simulink subsystem "Driver_Input"  (R2021b)
settings: Solver=VariableStepAuto  StartTime=0.0  StopTime=10.0  RelTol=1e-3
PostLoadFcn:
  | if any(exist('dsrtsu_mdlpostloadfcn', 'file') ~= 0), dsrtsu_mdlpostloadfcn('Execute', bdroot); end
libraries: simulink x9, dspstat3 x7, rtican x3, rti1401lib_adc_type4 x1
(part 1 of 2)
settings Model: DSRTSU_INTERNAL_RTI_VER=530  DSRTSU_INTERNAL_RTI_TYPE=rti1401  RTICANMMDATA=struct('GeneralSetupData',struct('modelroot','C:\Users\FEM\Documents\MATLAB\VCM_VehicleDynamicSim\VCMProgram\IO','generalsettings',struct('filesettings',struct('destfolder',struct('Name','RTICANMM_FILES','Check',1),'buildfolder',struct('Name','.','Check',1),'AbsDestfolder',struct('Name','C:\Users\FEM\Documents\MATLAB\VCM_VehicleDynamicSim\VCMProgram\IO\RTICANMM_FILES'),'AbsBuildfolder',struct('Name','C:\Users\FEM\Documents\MATLAB\VCM_VehicleDynamicSim\VCMProgram\IO'))),'options',struct('addpaths',1,'rmpaths',1,'addtrcexclusion',logical(1),'cannavigator',struct('checkmonitoring',0),'show_usrtrc',0,'use_usrtrc',0),'advanced',struct('options',ones(1,100)),'MPSetup',{{}},'RTI',struct('Type','GRT','Ver','','Date',''),'modelname','Driver_Input','block','Driver_Input'))  Creator=tsuyoshi  LastModifiedBy=FEM

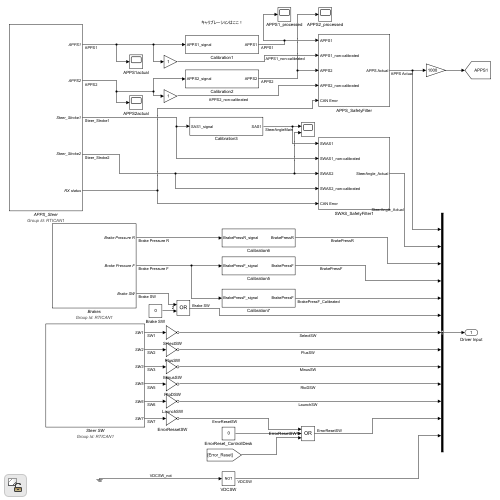
[thumbnail: Simulink's stored preview of the top-level diagram]
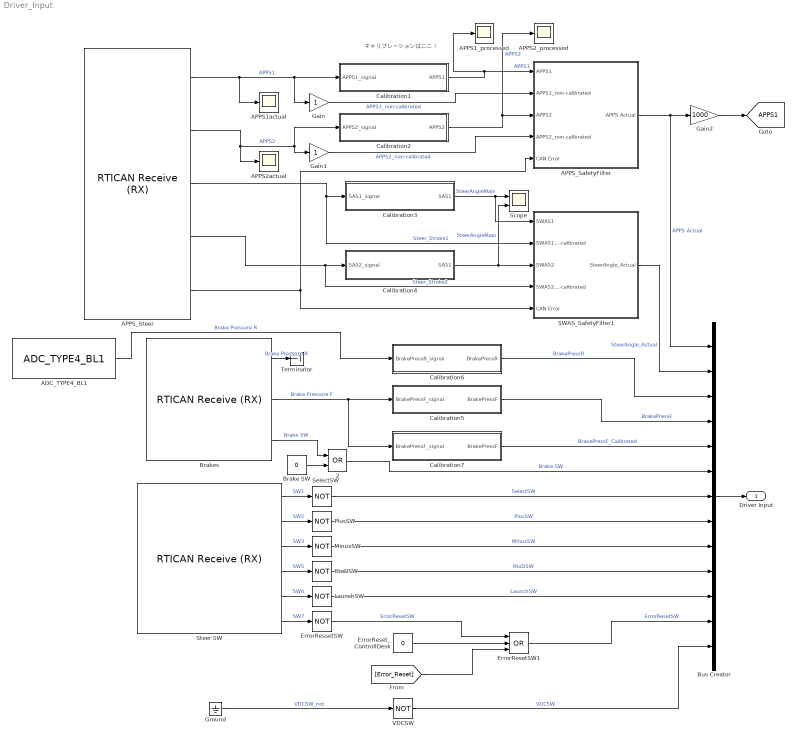
== system Driver_Input ==
  note: キャリブレーションはここ！
  2 : Logic  Operator=OR  AllPortsSameDT=off  OutDataTypeStr=boolean
  ADC_TYPE4_BL1 : rti1401lib_adc_type4/ADC_TYPE4_BL1  DSProperties=struct('RTI',struct('Version',uint32(2),'BlockType',struct('isSLSource',uint8(1),'isSLSink',uint8(1),'isHWSource',uint8(0),'isHWSink',uint8(1),'isSetup',uint8(0),'isInline',uint8(1),'isNonInline',uint8(0),'isInterrupt',uint8(0),'isChannelwise',uint8(1)),'IOBoardType',{{'DS1401','STD','ADCT4'}},'UnitType','ADC','Identifier','ADC','DialogType','ML','BlockSet','NONE','SlaveProcessor','NONE'))  RTIBlockInterface=struct('InputPortsActive',0,'InputPortsWidth',int32(1),'InputPortsDataType',{{'SS_BOOLEAN'}},'InputPortsName',{{'Continue'}},'OutputPortsActive',[1 0],'OutputPortsWidth',int32([1 1]),'OutputPortsDataType',{{'SS_DOUBLE','SS_UINT8'}},'OutputPortsName',{{'ADC','Status'}},'DialogFcn','rti1401stdadct4adcgui','SampleTime',{{-1}},'InitLevel',3,'IconTransparency','on','BlockDisplay',{{['ADC TP4\nModule: 1\nChannel: 6'],'center'}},'BlockName',struct('Token',{{'ADC_TYPE4_BL1'}}))  RTIBlockParameters=struct('ADCSWStartDisable',{{0,'OFF',[0 1]}},'ModuleNo',{{1,'OFF',[1 16]}},'ChannelNo',{{6,'OFF',[1 16]}},'ConversionMode',{{1,'OFF',[1 2]}},'SampleMode',{{1,'OFF',[1 2]}},'TriggerSource',{{1,'OFF',[1 5]}},'EdgePolarity',{{1,'OFF',[1 2]}},'ConversionTriggerSource',{{2,'OFF',[1 6]}},'ConversionEdgePolarity',{{1,'OFF',[1 2]}},'ConversionPeriod',{{'1e-06','OFF',[]}},'ConversionPeriodCheck',{{0,'OFF',[]}},'BurstTriggerSource',{{1,'OFF',[1 6]}},'BurstEdgePolarity',{{1,'OFF',[1 2]}},'BurstSize',{{'10','OFF',[]}},'BurstSizeCheck',{{0,'OFF',[]}},'DataSetOffset',{{'0','OFF',[]}},'DataSetOffsetCheck',{{0,'OFF',[]}},'DataSetLength',{{'1','OFF',[]}},'DataSetLengthCheck',{{0,'OFF',[]}},'ReadMode',{{1,'OFF',[1 2]}},'SampleTime',{{'-1','OFF',[-1 inf]}},'SampleTimeCheck',{{1,'OFF',[]}},'StatusPortEnable',{{0,'OFF',[0 1]}},'VoltageRange',{{2,'OFF',[1 2]}},'TLCFileName',{{'rti1401adc_t4_adc','OFF',[]}})  RTISFcnParameters=struct('ADCSWStartDisable','int32','ModuleNo','int32','ChannelNo','int16','ConversionMode','int16','SampleMode','int16','TriggerSource','int16','EdgePolarity','int16','ConversionTriggerSource','int16','ConversionEdgePolarity','int16','ConversionPeriod','double','BurstTriggerSource','int16','BurstEdgePolarity','int16','BurstSize','int16','DataSetOffset','int16','DataSetLength','int16','ReadMode','int16','SampleTime','double','StatusPortEnable','int16','VoltageRange','int16','TLCFileName','char')  RTIBlockParaDefault=struct('ADCSWStartDisable',0,'ModuleNo',1,'ChannelNo',1,'ConversionMode',1,'SampleMode',1,'TriggerSource',1,'EdgePolarity',1,'ConversionTriggerSource',2,'ConversionEdgePolarity',1,'ConversionPeriod',1e-6,'ConversionPeriodCheck',0,'BurstTriggerSource',1,'BurstEdgePolarity',1,'BurstSize',10,'BurstSizeCheck',0,'DataSetOffset',0,'DataSetOffsetCheck',0,'DataSetLength',1,'DataSetLengthCheck',0,'ReadMode',1,'SampleTime',-1,'SampleTimeCheck',1,'StatusPortEnable',0,'VoltageRange',1,'TLCFileName','rti1401adc_t4_adc')
  APPS1_processed : Scope
  APPS1actual : Scope
  APPS2_processed : Scope
  APPS2actual : Scope
  APPS_SafetyFilter : Subsystem
  APPS_Steer : rtican/RTICAN Receive (RX)   Reserved1=[]  Reserved2=[]  Reserved3=[]  Reserved4=[]  SfcnMessage=[]  Msg_Struct=[]  BoardTypeNo=[]  BoardNo=[]  ChannelNo=[]  Parameters=[]  DialogFcn=[]  UnitName=[]  Revision=[]  UnitValues=[]  DSProperties=struct('RTI',struct('Version',uint32(5),'BlockType',struct('isSLSource',uint8(1),'isSLSink',uint8(1),'isHWSource',uint8(0),'isHWSink',uint8(0),'isSetup',uint8(0),'isInline',uint8(1),'isNonInline',uint8(0),'isInterrupt',uint8(0),'isChannelwise',uint8(0)),'IOBoardType','RTICAN','UnitType','MESSAGE','Identifier','RX','DialogType','MSVC','BlockSet','RTICAN','SlaveProcessor','CAN'))  RTIBlockInterface=struct('OutputPortsWidth',int32([1 1 1 1 1]),'OutputPortsActive',[1 1 1 1 1],'OutputPortsName',{{'APPS1','APPS2','Steer_Stroke1','Steer_Stroke2',['RX status']}},'OutputPortsDataType',{{'SS_DOUBLE','SS_DOUBLE','SS_DOUBLE','SS_DOUBLE','SS_DOUBLE'}},'OutputPortsLabel',{{'APPS1','APPS2','Steer_Stroke1','Steer_Stroke2',''}},'OutputPortsLabelMode','ON','InputPortsWidth',int32(0),'InputPortsActive',0,'DialogFcn','rtican_message_interface_gui','BlockDisplay',{{'','center'}},'IconTransparency','on','ParameterTunableNames',{{}},'InitLevel',3,'BlockName',struct('Token',{{'APPS_Steer'}}),'SampleTime',{{0.01}},'TriggerPort',{{'none'}},'EnablePort',{{'none'}})  RTIBlockParameters=struct('BoardTypeNo',{{1,'OFF',[]}},'BoardNo',{{1,'ON',[1 16]}},'ChannelNo',{{1,'ON',[1 2]}},'Parameters',{{struct('DataFileSupport',struct('DataFileSelectedMaster',0,'DataFileSelectedLocal',0,'DataFileName',['<no datafile support>|'],'DataFileDate','','SelectedFile',['<no file selected>']),'Options',struct('StatusSelected',1,'TimeSelected',0,'DeltaTimeSelected',0,'BytePortSelected',0,'MessageLengthSelected',0,'TriggerPort',struct('Selected',0,'TriggerType',0),'UserCoding',struct('Selected',0,'InterfaceFile','UserDecodingFile','FcnName','UserDecodeFcn','InportSelected',0,'InportWidth',1,'OutportSelected',0,'OutportWidth',1),'EnablePortSelected',0,'SignalOnPortnameSelected',1,'UseRXService',0),'Message',struct('MsgOnBlocknameSelected',1,'MsgName','APPS_Steer','MsgIdFormat',0,'MsgId',513,'MsgLength',8,'NumSignals',4,'SampleTime',0.01,'Signal',struct('SgnName',{'APPS1','APPS2','Steer_Stroke1','Steer_Stroke2'},'SgnStartBit',{0,16,32,48},'SgnLength',{16,16,16,16},'SgnType',{0,0,0,0},'ModeValue',{-1,-1,-1,-1},'DataType',{0,0,0,0},'ByteLayout',{0,0,0,0},'Factor',{1,1,1,1},'Offset',{0,0,0,0},'SgnComment',{{''},{''},{''},{''}},'SgnUnit',{'','','',''},'Min',{0,0,0,0},'Max',{0,0,0,0},'SLDataType',{'SS_DOUBLE','SS_DOUBLE','SS_DOUBLE','SS_DOUBLE'}),'MsgIdNumFormat',1,'MsgComment',{{''}}),'Version',1.2,'general',struct('isFromLib',0)),'OFF',[]}},'GroupId',{{struct('Group',{{'RTICAN'}},'No',1,'Behavior',{{'NAMECHANGE'}},'BlockType',{{'SINK'}},'NameChangeFlag',0),'OFF',[]}},'SFcnRTICANMessage',{{struct('MsgType','RX','SFcnPortType','Scalar','MsgName','APPS_Steer','MsgIdFormat','STD','MsgId',513,'MsgLength',8,'NumSignals',4,'SampleTime',0.01,'Signal',struct('SgnName',{'APPS1','APPS2','Steer_Stroke1','Steer_Stroke2'},'SgnStartBit',{0,16,32,48},'SgnLength',{16,16,16,16},'SgnType',{'standard','standard','standard','standard'},'ModeValue',{-1,-1,-1,-1},'DataType',{['unsigned int'],['unsigned int'],['unsigned int'],['unsigned int']},'ByteLayout',{['little endian'],['little endian'],['little endian'],['little endian']},'Factor',{1,1,1,1},'Offset',{0,0,0,0},'SLDataType',{'SS_DOUBLE','SS_DOUBLE','SS_DOUBLE','SS_DOUBLE'}),'StatusSelected','yes','TimeSelected','no','DeltaTimeSelected','no','BytePortSelected','no','MessageLengthSelected','no','TriggerPort',struct('Selected','no','TriggerType',0),'UserCoding',struct('Selected','no','InterfaceFile','UserDecodingFile','FcnName','UserDecodeFcn','InportSelected','no','InportWidth',1,'OutportSelected','no','OutportWidth',1),'EnablePortSelected','no','UseRXService','no','BoardType','DS1','BoardNo',1,'ControllerNo',1),'OFF',[]}},'TLCFileName',{{'rtican_rx_message','OFF',[]}})  RTISFcnParameters=struct('SFcnRTICANMessage','struct','TLCFileName','char')  RTIBlockParaDefault=struct('BoardTypeNo',4302,'BoardNo',1,'ChannelNo',1,'Parameters',struct('DataFileSupport',struct('DataFileSelectedMaster',0,'DataFileSelectedLocal',0,'DataFileName','','DataFileDate','','SelectedFile',['<no file selected>']),'Options',struct('StatusSelected',1,'TimeSelected',1,'DeltaTimeSelected',1,'BytePortSelected',0,'MessageLengthSelected',0,'TriggerPort',struct('Selected',0,'TriggerType','rising'),'UserCoding',struct('Selected',0,'InterfaceFile','UserDecodingFile','FcnName','UserDecodeFcn','InportSelected',0,'InportWidth',1,'OutportSelected',0,'OutportWidth',1),'EnablePortSelected',0,'SignalOnPortnameSelected',1,'UseRXService',0),'Message',struct('MsgOnBlocknameSelected',0,'MsgName',['RX Message'],'MsgIdFormat',0,'MsgId',100,'MsgLength',8,'NumSignals',1,'SampleTime',-1,'Signal',struct('SgnName',['RX signal'],'SgnStartBit',0,'SgnLength',8,'SgnType',0,'ModeValue',-1,'DataType',0,'SLDataType','SS_DOUBLE','ByteLayout',0,'Factor',1,'Offset',0,'Min',0,'Max',255,'SgnComment',{{}},'SgnUnit',''),'MsgIdNumFormat',0,'MsgComment',{{''}}),'Version',1.2,'general',struct('isFromLib',1)),'GroupId',struct('Group',{{'RTICAN'}},'No',1,'Behavior',{{'NAMECHANGE'}},'BlockType',{{'SINK'}},'NameChangeFlag',0),'SFcnRTICANMessage',struct('MsgType','RX','MsgName',['RX Message'],'MsgIdFormat','STD','MsgId',100,'MsgLength',8,'NumSignals',1,'SampleTime',-1,'Signal',struct('SgnName',['RX signal'],'SgnStartBit',0,'SgnLength',8,'SgnType','standard','ModeValue',-1,'DataType',['unsigned int'],'ByteLayout',['little endian'],'SLDataType','SS_DOUBLE','Factor',1,'Offset',0),'StatusSelected','yes','TimeSelected','yes','DeltaTimeSelected','yes','BytePortSelected','no','MessageLengthSelected','no','EnablePortSelected','no','UserCoding',struct('Selected','no','InterfaceFile','UserDecodingFile','FcnName','UserDecodeFcn','InportSelected','no','InportWidth',1,'OutportSelected','no','OutportWidth',1),'TriggerPort',struct('Selected','no','TriggerType','rising'),'UseRXService','no','BoardType','DS4302','BoardNo',1,'ControllerNo',1,'SFcnPortType','Scalar'),'TLCFileName','rtican_rx_message')
      settings: AttributesFormatString=Group Id: RTICAN1\n  SourceProductName=dSPACE RTI CAN Blockset
  Brake SW : Constant  Value=0
  Brakes : rtican/RTICAN Receive (RX)   Reserved1=[]  Reserved2=[]  Reserved3=[]  Reserved4=[]  SfcnMessage=[]  Msg_Struct=[]  BoardTypeNo=[]  BoardNo=[]  ChannelNo=[]  Parameters=[]  DialogFcn=[]  UnitName=[]  Revision=[]  UnitValues=[]  DSProperties=struct('RTI',struct('Version',uint32(5),'BlockType',struct('isSLSource',uint8(1),'isSLSink',uint8(1),'isHWSource',uint8(0),'isHWSink',uint8(0),'isSetup',uint8(0),'isInline',uint8(1),'isNonInline',uint8(0),'isInterrupt',uint8(0),'isChannelwise',uint8(0)),'IOBoardType','RTICAN','UnitType','MESSAGE','Identifier','RX','DialogType','MSVC','BlockSet','RTICAN','SlaveProcessor','CAN'))  RTIBlockInterface=struct('OutputPortsWidth',int32([1 1 1]),'OutputPortsActive',[1 1 1],'OutputPortsName',{{['Brake Pressure R'],['Brake Pressure F'],['Brake SW']}},'OutputPortsDataType',{{'SS_DOUBLE','SS_DOUBLE','SS_DOUBLE'}},'OutputPortsLabel',{{['Brake Pressure R'],['Brake Pressure F'],['Brake SW']}},'OutputPortsLabelMode','ON','InputPortsWidth',int32(0),'InputPortsActive',0,'DialogFcn','rtican_message_interface_gui','BlockDisplay',{{'','center'}},'IconTransparency','on','ParameterTunableNames',{{}},'InitLevel',3,'BlockName',struct('Token',{{'Brakes'}}),'SampleTime',{{0.01}},'TriggerPort',{{'none'}},'EnablePort',{{'none'}})  RTIBlockParameters=struct('BoardTypeNo',{{1,'OFF',[]}},'BoardNo',{{1,'ON',[1 16]}},'ChannelNo',{{1,'ON',[1 2]}},'Parameters',{{struct('DataFileSupport',struct('DataFileSelectedMaster',0,'DataFileSelectedLocal',0,'DataFileName',['<no datafile support>|'],'DataFileDate','','SelectedFile',['<no file selected>']),'Options',struct('StatusSelected',0,'TimeSelected',0,'DeltaTimeSelected',0,'BytePortSelected',0,'MessageLengthSelected',0,'TriggerPort',struct('Selected',0,'TriggerType',0),'UserCoding',struct('Selected',0,'InterfaceFile','UserDecodingFile','FcnName','UserDecodeFcn','InportSelected',0,'InportWidth',1,'OutportSelected',0,'OutportWidth',1),'EnablePortSelected',0,'SignalOnPortnameSelected',1,'UseRXService',0),'Message',struct('MsgOnBlocknameSelected',1,'MsgName','Brakes','MsgIdFormat',0,'MsgId',514,'MsgLength',8,'NumSignals',3,'SampleTime',0.01,'Signal',struct('SgnName',{['Brake Pressure R'],['Brake Pressure F'],['Brake SW']},'SgnStartBit',{0,16,32},'SgnLength',{16,16,8},'SgnType',{0,0,0},'ModeValue',{-1,-1,-1},'DataType',{0,0,0},'ByteLayout',{0,0,0},'Factor',{1,1,1},'Offset',{0,0,0},'SgnComment',{{''},{''},{''}},'SgnUnit',{'','',''},'Min',{0,0,0},'Max',{0,0,0},'SLDataType',{'SS_DOUBLE','SS_DOUBLE','SS_DOUBLE'}),'MsgIdNumFormat',1,'MsgComment',{{''}}),'Version',1.2,'general',struct('isFromLib',0)),'OFF',[]}},'GroupId',{{struct('Group',{{'RTICAN'}},'No',1,'Behavior',{{'NAMECHANGE'}},'BlockType',{{'SINK'}},'NameChangeFlag',0),'OFF',[]}},'SFcnRTICANMessage',{{struct('MsgType','RX','SFcnPortType','Scalar','MsgName','Brakes','MsgIdFormat','STD','MsgId',514,'MsgLength',8,'NumSignals',3,'SampleTime',0.01,'Signal',struct('SgnName',{['Brake Pressure R'],['Brake Pressure F'],['Brake SW']},'SgnStartBit',{0,16,32},'SgnLength',{16,16,8},'SgnType',{'standard','standard','standard'},'ModeValue',{-1,-1,-1},'DataType',{['unsigned int'],['unsigned int'],['unsigned int']},'ByteLayout',{['little endian'],['little endian'],['little endian']},'Factor',{1,1,1},'Offset',{0,0,0},'SLDataType',{'SS_DOUBLE','SS_DOUBLE','SS_DOUBLE'}),'StatusSelected','no','TimeSelected','no','DeltaTimeSelected','no','BytePortSelected','no','MessageLengthSelected','no','TriggerPort',struct('Selected','no','TriggerType',0),'UserCoding',struct('Selected','no','InterfaceFile','UserDecodingFile','FcnName','UserDecodeFcn','InportSelected','no','InportWidth',1,'OutportSelected','no','OutportWidth',1),'EnablePortSelected','no','UseRXService','no','BoardType','DS1','BoardNo',1,'ControllerNo',1),'OFF',[]}},'TLCFileName',{{'rtican_rx_message','OFF',[]}})  RTISFcnParameters=struct('SFcnRTICANMessage','struct','TLCFileName','char')  RTIBlockParaDefault=struct('BoardTypeNo',4302,'BoardNo',1,'ChannelNo',1,'Parameters',struct('DataFileSupport',struct('DataFileSelectedMaster',0,'DataFileSelectedLocal',0,'DataFileName','','DataFileDate','','SelectedFile',['<no file selected>']),'Options',struct('StatusSelected',1,'TimeSelected',1,'DeltaTimeSelected',1,'BytePortSelected',0,'MessageLengthSelected',0,'TriggerPort',struct('Selected',0,'TriggerType','rising'),'UserCoding',struct('Selected',0,'InterfaceFile','UserDecodingFile','FcnName','UserDecodeFcn','InportSelected',0,'InportWidth',1,'OutportSelected',0,'OutportWidth',1),'EnablePortSelected',0,'SignalOnPortnameSelected',1,'UseRXService',0),'Message',struct('MsgOnBlocknameSelected',0,'MsgName',['RX Message'],'MsgIdFormat',0,'MsgId',100,'MsgLength',8,'NumSignals',1,'SampleTime',-1,'Signal',struct('SgnName',['RX signal'],'SgnStartBit',0,'SgnLength',8,'SgnType',0,'ModeValue',-1,'DataType',0,'SLDataType','SS_DOUBLE','ByteLayout',0,'Factor',1,'Offset',0,'Min',0,'Max',255,'SgnComment',{{}},'SgnUnit',''),'MsgIdNumFormat',0,'MsgComment',{{''}}),'Version',1.2,'general',struct('isFromLib',1)),'GroupId',struct('Group',{{'RTICAN'}},'No',1,'Behavior',{{'NAMECHANGE'}},'BlockType',{{'SINK'}},'NameChangeFlag',0),'SFcnRTICANMessage',struct('MsgType','RX','MsgName',['RX Message'],'MsgIdFormat','STD','MsgId',100,'MsgLength',8,'NumSignals',1,'SampleTime',-1,'Signal',struct('SgnName',['RX signal'],'SgnStartBit',0,'SgnLength',8,'SgnType','standard','ModeValue',-1,'DataType',['unsigned int'],'ByteLayout',['little endian'],'SLDataType','SS_DOUBLE','Factor',1,'Offset',0),'StatusSelected','yes','TimeSelected','yes','DeltaTimeSelected','yes','BytePortSelected','no','MessageLengthSelected','no','EnablePortSelected','no','UserCoding',struct('Selected','no','InterfaceFile','UserDecodingFile','FcnName','UserDecodeFcn','InportSelected','no','InportWidth',1,'OutportSelected','no','OutportWidth',1),'TriggerPort',struct('Selected','no','TriggerType','rising'),'UseRXService','no','BoardType','DS4302','BoardNo',1,'ControllerNo',1,'SFcnPortType','Scalar'),'TLCFileName','rtican_rx_message')
      settings: AttributesFormatString=Group Id: RTICAN1\n  SourceProductName=dSPACE RTI CAN Blockset
  Bus Creator : BusCreator  Inputs=13
  Calibration1 : Subsystem
  Calibration2 : Subsystem
  Calibration3 : Subsystem
  Calibration4 : Subsystem
  Calibration5 : Subsystem
  Calibration6 : Subsystem
  Calibration7 : Subsystem
  ErrorResetSW1 : Logic  Operator=OR  Inputs=3  AllPortsSameDT=off  OutDataTypeStr=boolean
  ErrorReset_ControllDesk : Constant  Value=0
  ErrorRessetSW : Logic  Operator=NOT  IconShape=distinctive  AllPortsSameDT=off  OutDataTypeStr=boolean
  Gain : Gain
  Gain1 : Gain
  Gain2 : Gain  Gain=1000
  Ground : Ground
  LaunchSW : Logic  Operator=NOT  IconShape=distinctive  AllPortsSameDT=off  OutDataTypeStr=boolean
  MinusSW : Logic  Operator=NOT  IconShape=distinctive  AllPortsSameDT=off  OutDataTypeStr=boolean
  PlusSW : Logic  Operator=NOT  IconShape=distinctive  AllPortsSameDT=off  OutDataTypeStr=boolean
  RtoDSW : Logic  Operator=NOT  IconShape=distinctive  AllPortsSameDT=off  OutDataTypeStr=boolean
  SWAS_SafetyFilter1 : Subsystem
  Scope : Scope  NumInputPorts=2
  SelectSW : Logic  Operator=NOT  IconShape=distinctive  AllPortsSameDT=off  OutDataTypeStr=boolean
  Steer SW : rtican/RTICAN Receive (RX)   Reserved1=[]  Reserved2=[]  Reserved3=[]  Reserved4=[]  SfcnMessage=[]  Msg_Struct=[]  BoardTypeNo=[]  BoardNo=[]  ChannelNo=[]  Parameters=[]  DialogFcn=[]  UnitName=[]  Revision=[]  UnitValues=[]  DSProperties=struct('RTI',struct('Version',uint32(5),'BlockType',struct('isSLSource',uint8(1),'isSLSink',uint8(1),'isHWSource',uint8(0),'isHWSink',uint8(0),'isSetup',uint8(0),'isInline',uint8(1),'isNonInline',uint8(0),'isInterrupt',uint8(0),'isChannelwise',uint8(0)),'IOBoardType','RTICAN','UnitType','MESSAGE','Identifier','RX','DialogType','MSVC','BlockSet','RTICAN','SlaveProcessor','CAN'))  RTIBlockInterface=struct('OutputPortsWidth',int32([1 1 1 1 1 1]),'OutputPortsActive',[1 1 1 1 1 1],'OutputPortsName',{{'SW1','SW2','SW3','SW5','SW6','SW7'}},'OutputPortsDataType',{{'SS_DOUBLE','SS_DOUBLE','SS_DOUBLE','SS_DOUBLE','SS_DOUBLE','SS_DOUBLE'}},'OutputPortsLabel',{{'SW1','SW2','SW3','SW5','SW6','SW7'}},'OutputPortsLabelMode','ON','InputPortsWidth',int32(0),'InputPortsActive',0,'DialogFcn','rtican_message_interface_gui','BlockDisplay',{{'','center'}},'IconTransparency','on','ParameterTunableNames',{{}},'InitLevel',3,'BlockName',struct('Token',{{'Brakes'}}),'SampleTime',{{0.1}},'TriggerPort',{{'none'}},'EnablePort',{{'none'}})  RTIBlockParameters=struct('BoardTypeNo',{{1,'OFF',[]}},'BoardNo',{{1,'ON',[1 16]}},'ChannelNo',{{1,'ON',[1 2]}},'Parameters',{{struct('DataFileSupport',struct('DataFileSelectedMaster',0,'DataFileSelectedLocal',0,'DataFileName',['<no datafile support>|'],'DataFileDate','','SelectedFile',['<no file selected>']),'Options',struct('StatusSelected',0,'TimeSelected',0,'DeltaTimeSelected',0,'BytePortSelected',0,'MessageLengthSelected',0,'TriggerPort',struct('Selected',0,'TriggerType',0),'UserCoding',struct('Selected',0,'InterfaceFile','UserDecodingFile','FcnName','UserDecodeFcn','InportSelected',0,'InportWidth',1,'OutportSelected',0,'OutportWidth',1),'EnablePortSelected',0,'SignalOnPortnameSelected',1,'UseRXService',0),'Message',struct('MsgOnBlocknameSelected',1,'MsgName',['Steer SW'],'MsgIdFormat',0,'MsgId',512,'MsgLength',1,'NumSignals',6,'SampleTime',0.1,'Signal',struct('SgnName',{'SW1','SW2','SW3','SW5','SW6','SW7'},'SgnStartBit',{0,1,2,3,4,5},'SgnLength',{1,1,1,1,1,1},'SgnType',{0,0,0,0,0,0},'ModeValue',{-1,-1,-1,-1,-1,-1},'DataType',{0,0,0,0,0,0},'ByteLayout',{0,0,0,0,0,0},'Factor',{1,1,1,1,1,1},'Offset',{0,0,0,0,0,0},'SgnComment',{{''},{''},{''},{''},{''},{''}},'SgnUnit',{'','','','','',''},'Min',{0,0,0,0,0,0},'Max',{0,0,0,0,0,0},'SLDataType',{'SS_DOUBLE','SS_DOUBLE','SS_DOUBLE','SS_DOUBLE','SS_DOUBLE','SS_DOUBLE'}),'MsgIdNumFormat',1,'MsgComment',{{''}}),'Version',1.2,'general',struct('isFromLib',0)),'OFF',[]}},'GroupId',{{struct('Group',{{'RTICAN'}},'No',1,'Behavior',{{'NAMECHANGE'}},'BlockType',{{'SINK'}},'NameChangeFlag',0),'OFF',[]}},'SFcnRTICANMessage',{{struct('MsgType','RX','SFcnPortType','Scalar','MsgName',['Steer SW'],'MsgIdFormat','STD','MsgId',512,'MsgLength',1,'NumSignals',6,'SampleTime',0.1,'Signal',struct('SgnName',{'SW1','SW2','SW3','SW5','SW6','SW7'},'SgnStartBit',{0,1,2,3,4,5},'SgnLength',{1,1,1,1,1,1},'SgnType',{'standard','standard','standard','standard','standard','standard'},'ModeValue',{-1,-1,-1,-1,-1,-1},'DataType',{['unsigned int'],['unsigned int'],['unsigned int'],['unsigned int'],['unsigned int'],['unsigned int']},'ByteLayout',{['little endian'],['little endian'],['little endian'],['little endian'],['little endian'],['little endian']},'Factor',{1,1,1,1,1,1},'Offset',{0,0,0,0,0,0},'SLDataType',{'SS_DOUBLE','SS_DOUBLE','SS_DOUBLE','SS_DOUBLE','SS_DOUBLE','SS_DOUBLE'}),'StatusSelected','no','TimeSelected','no','DeltaTimeSelected','no','BytePortSelected','no','MessageLengthSelected','no','TriggerPort',struct('Selected','no','TriggerType',0),'UserCoding',struct('Selected','no','InterfaceFile','UserDecodingFile','FcnName','UserDecodeFcn','InportSelected','no','InportWidth',1,'OutportSelected','no','OutportWidth',1),'EnablePortSelected','no','UseRXService','no','BoardType','DS1','BoardNo',1,'ControllerNo',1),'OFF',[]}},'TLCFileName',{{'rtican_rx_message','OFF',[]}})  RTISFcnParameters=struct('SFcnRTICANMessage','struct','TLCFileName','char')  RTIBlockParaDefault=struct('BoardTypeNo',4302,'BoardNo',1,'ChannelNo',1,'Parameters',struct('DataFileSupport',struct('DataFileSelectedMaster',0,'DataFileSelectedLocal',0,'DataFileName','','DataFileDate','','SelectedFile',['<no file selected>']),'Options',struct('StatusSelected',1,'TimeSelected',1,'DeltaTimeSelected',1,'BytePortSelected',0,'MessageLengthSelected',0,'TriggerPort',struct('Selected',0,'TriggerType','rising'),'UserCoding',struct('Selected',0,'InterfaceFile','UserDecodingFile','FcnName','UserDecodeFcn','InportSelected',0,'InportWidth',1,'OutportSelected',0,'OutportWidth',1),'EnablePortSelected',0,'SignalOnPortnameSelected',1,'UseRXService',0),'Message',struct('MsgOnBlocknameSelected',0,'MsgName',['RX Message'],'MsgIdFormat',0,'MsgId',100,'MsgLength',8,'NumSignals',1,'SampleTime',-1,'Signal',struct('SgnName',['RX signal'],'SgnStartBit',0,'SgnLength',8,'SgnType',0,'ModeValue',-1,'DataType',0,'SLDataType','SS_DOUBLE','ByteLayout',0,'Factor',1,'Offset',0,'Min',0,'Max',255,'SgnComment',{{}},'SgnUnit',''),'MsgIdNumFormat',0,'MsgComment',{{''}}),'Version',1.2,'general',struct('isFromLib',1)),'GroupId',struct('Group',{{'RTICAN'}},'No',1,'Behavior',{{'NAMECHANGE'}},'BlockType',{{'SINK'}},'NameChangeFlag',0),'SFcnRTICANMessage',struct('MsgType','RX','MsgName',['RX Message'],'MsgIdFormat','STD','MsgId',100,'MsgLength',8,'NumSignals',1,'SampleTime',-1,'Signal',struct('SgnName',['RX signal'],'SgnStartBit',0,'SgnLength',8,'SgnType','standard','ModeValue',-1,'DataType',['unsigned int'],'ByteLayout',['little endian'],'SLDataType','SS_DOUBLE','Factor',1,'Offset',0),'StatusSelected','yes','TimeSelected','yes','DeltaTimeSelected','yes','BytePortSelected','no','MessageLengthSelected','no','EnablePortSelected','no','UserCoding',struct('Selected','no','InterfaceFile','UserDecodingFile','FcnName','UserDecodeFcn','InportSelected','no','InportWidth',1,'OutportSelected','no','OutportWidth',1),'TriggerPort',struct('Selected','no','TriggerType','rising'),'UseRXService','no','BoardType','DS4302','BoardNo',1,'ControllerNo',1,'SFcnPortType','Scalar'),'TLCFileName','rtican_rx_message')
      settings: AttributesFormatString=Group Id: RTICAN1\n  SourceProductName=dSPACE RTI CAN Blockset
  Terminator : Terminator
  VDCSW : Logic  Operator=NOT  AllPortsSameDT=off  OutDataTypeStr=boolean
  Driver Input : Outport  VectorParamsAs1DForOutWhenUnconnected=off
  tag scope: APPS1=global
  wires:
  APPS_Steer/1 -> Calibration1/1(APPS1_signal), Gain/1, APPS1actual/1  "APPS1"
  APPS_Steer/2 -> Gain1/1, Calibration2/1(APPS2_signal), APPS2actual/1  "APPS2"
  APPS_Steer/3 -> SWAS_SafetyFilter1/2(SWAS1_non-calibrated), Calibration3/1(SAS1_signal)  "Steer_Stroke1"
  APPS_Steer/4 -> Calibration4/1(SAS2_signal), SWAS_SafetyFilter1/4(SWAS2_non-calibrated)  "Steer_Stroke2"
  Brakes/2 -> Calibration5/1(BrakePressF_signal), Calibration7/1(BrakePressF_signal)  "Brake Pressure F"
  ADC_TYPE4_BL1/1 -> Calibration6/1(BrakePressR_signal)  "Brake Pressure R"
  Calibration3/1(SAS1) -> Scope/1, SWAS_SafetyFilter1/1(SWAS1)  "SteerAngleMain"
  Calibration5/1(BrakePressF) -> Bus Creator/4  "BrakePressF"
  Calibration6/1(BrakePressR) -> Bus Creator/3  "BrakePressR"
  Bus Creator/1 -> Driver Input/1
  RtoDSW/1 -> Bus Creator/10  "RtoDSW"
  LaunchSW/1 -> Bus Creator/11  "LaunchSW"
  ErrorResetSW1/1 -> Bus Creator/12  "ErrorResetSW"
  VDCSW/1 -> Bus Creator/13  "VDCSW"
  Ground/1 -> VDCSW/1  "VDCSW_not"
  ErrorRessetSW/1 -> ErrorResetSW1/1  "ErrorResetSW"
  ErrorReset_ControllDesk/1 -> ErrorResetSW1/2
  Calibration1/1(APPS1) -> APPS1_processed/1, APPS_SafetyFilter/1(APPS1)  "APPS1"
  Calibration2/1(APPS2) -> APPS2_processed/1, APPS_SafetyFilter/3(APPS2)  "APPS2"
  Gain/1 -> APPS_SafetyFilter/2(APPS1_non-calibrated)  "APPS1_non-calibrated"
  Gain1/1 -> APPS_SafetyFilter/4(APPS2_non-calibrated)  "APPS2_non-calibrated"
  APPS_SafetyFilter/1(APPS Actual) -> Bus Creator/1, Gain2/1  "APPS Actual"
  SWAS_SafetyFilter1/1(SteerAngle_Actual) -> Bus Creator/2  "SteerAngle_Actual"
  Steer SW/1 -> SelectSW/1  "SW1"
  Steer SW/2 -> PlusSW/1  "SW2"
  Steer SW/3 -> MinusSW/1  "SW3"
  SelectSW/1 -> Bus Creator/7  "SelectSW"
  PlusSW/1 -> Bus Creator/8  "PlusSW"
  MinusSW/1 -> Bus Creator/9  "MinusSW"
  Steer SW/4 -> RtoDSW/1  "SW5"
  Steer SW/5 -> LaunchSW/1  "SW6"
  Steer SW/6 -> ErrorRessetSW/1  "SW7"
  2/1 -> Bus Creator/6  "Brake SW"
  Gain2/1 -> [APPS1]
  APPS_Steer/5 -> APPS_SafetyFilter/5(CAN Error), SWAS_SafetyFilter1/5(CAN Error)
  Calibration7/1(BrakePressF) -> Bus Creator/5  "BrakePressF_Calibrated"
  [Error_Reset] -> ErrorResetSW1/3
  Brakes/3 -> 2/1  "Brake SW"
  Brake SW/1 -> 2/2
  Brakes/1 -> Terminator/1  "Brake Pressure R"
  Calibration4/1(SAS1) -> SWAS_SafetyFilter1/3(SWAS2), Scope/2  "SteerAngleMain"

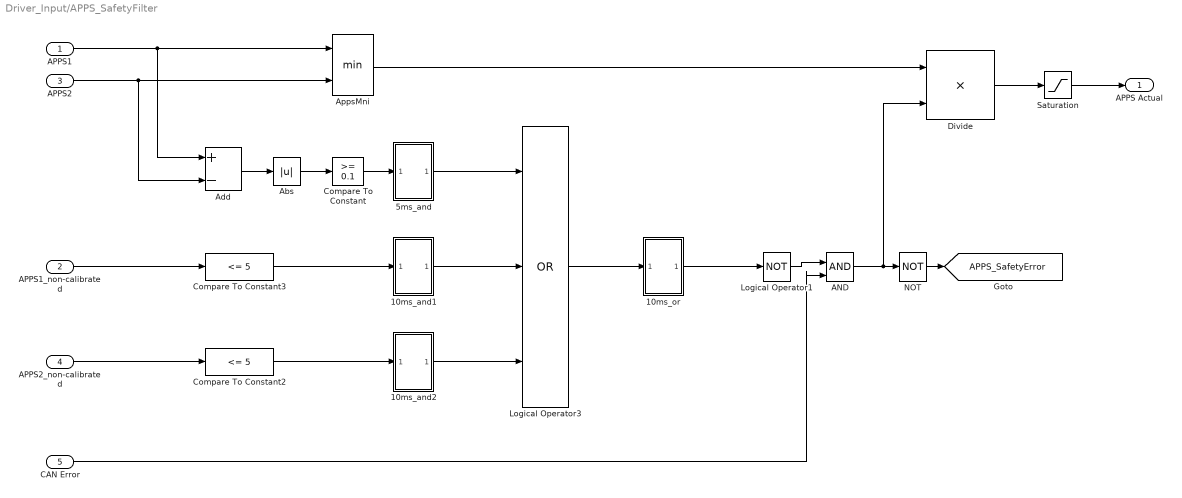
== system Driver_Input/APPS_SafetyFilter ==
  APPS1 : Inport
  APPS1_non-calibrated : Inport  Port=2
  APPS2 : Inport  Port=3
  APPS2_non-calibrated : Inport  Port=4
  CAN Error : Inport  Port=5
  10ms_and1 : Subsystem
  10ms_and2 : Subsystem
  10ms_or : Subsystem
  5ms_and : Subsystem
  AND : Logic  IconShape=distinctive  AllPortsSameDT=off  OutDataTypeStr=boolean
  Abs : Abs
  Add : Sum  Inputs=+-
  AppsMni : MinMax  Inputs=2
  Compare To Constant : simulink/Logic and Bit Operations/Compare To Constant  relop=>=  const=0.1  OutDataTypeStr=boolean
  Compare To Constant2 : simulink/Logic and Bit Operations/Compare To Constant  relop=<=  const=5  OutDataTypeStr=boolean
  Compare To Constant3 : simulink/Logic and Bit Operations/Compare To Constant  relop=<=  const=5  OutDataTypeStr=boolean
  Divide : Product  Inputs=**
  Logical Operator1 : Logic  Operator=NOT  AllPortsSameDT=off  OutDataTypeStr=boolean
  Logical Operator3 : Logic  Operator=OR  Inputs=3  AllPortsSameDT=off  OutDataTypeStr=boolean
  NOT : Logic  Operator=NOT  IconShape=distinctive  AllPortsSameDT=off  OutDataTypeStr=boolean
  Saturation : Saturate  UpperLimit=1  LowerLimit=0
  APPS Actual : Outport  VectorParamsAs1DForOutWhenUnconnected=off
  tag scope: APPS_SafetyError=global
  wires:
  NOT/1 -> [APPS_SafetyError]
  Logical Operator1/1 -> AND/1
  10ms_or/1(Out1) -> Logical Operator1/1
  CAN Error/1 -> AND/2
  10ms_and2/1(Out1) -> Logical Operator3/3
  10ms_and1/1(Out1) -> Logical Operator3/2
  Logical Operator3/1 -> 10ms_or/1(In1)
  APPS2_non-calibrated/1 -> Compare To Constant2/1
  Compare To Constant2/1 -> 10ms_and2/1(In1)
  Compare To Constant3/1 -> 10ms_and1/1(In1)
  APPS1_non-calibrated/1 -> Compare To Constant3/1
  5ms_and/1(Out1) -> Logical Operator3/1
  Compare To Constant/1 -> 5ms_and/1(In1)
  APPS2/1 -> AppsMni/2, Add/2
  APPS1/1 -> AppsMni/1, Add/1
  Saturation/1 -> APPS Actual/1
  AppsMni/1 -> Divide/1
  Divide/1 -> Saturation/1
  AND/1 -> NOT/1, Divide/2
  Add/1 -> Abs/1
  Abs/1 -> Compare To Constant/1

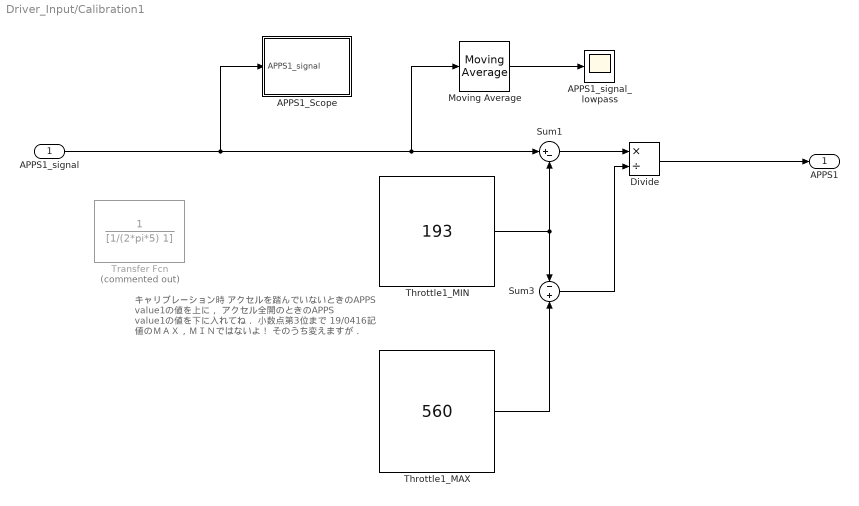
== system Driver_Input/Calibration1 ==
  note: キャリブレーション時
      | アクセルを踏んでいないときのAPPS value1の値を上に，
      | アクセル全開のときのAPPS value1の値を下に入れてね．
      | 小数点第3位まで
      |
      | 19/0416記
      | 値のＭＡＸ，ＭＩＮではないよ！
      | そのうち変えますが．
  APPS1_signal : Inport
  APPS1_Scope : Subsystem
  APPS1_signal_lowpass : Scope
  Divide : Product  Inputs=*/  RndMeth=Zero  SaturateOnIntegerOverflow=on
  Moving Average : dspstat3/Moving Average  Method=Sliding window  ForgettingFactorPort=off  SpecifyWindowLength=on  WindowLength=1000  ForgettingFactor=0.9  SimulateUsing=Code generation
  Sum1 : Sum  Inputs=|+-
  Sum3 : Sum  Inputs=-+
  Throttle1_MAX : Constant  Value=560  OutDataTypeStr=double
  Throttle1_MIN : Constant  Value=193  OutDataTypeStr=double
  Transfer Fcn : TransferFcn  Commented=on  Denominator=[1/(2*pi*5) 1]
  APPS1 : Outport  VectorParamsAs1DForOutWhenUnconnected=off
  wires:
  Moving Average/1 -> APPS1_signal_lowpass/1
  APPS1_signal/1 -> APPS1_Scope/1(APPS1_signal), Sum1/1, Moving Average/1
  Divide/1 -> APPS1/1
  Throttle1_MAX/1 -> Sum3/2
  Sum1/1 -> Divide/1
  Sum3/1 -> Divide/2
  Throttle1_MIN/1 -> Sum3/1, Sum1/2

== system Driver_Input/Calibration2 ==
  note: キャリブレーション時
      | アクセルを踏んでいないときのAPPS value２の値を上に，
      | アクセル全開のときのAPPS value２の値を下に入れてね．
      | 小数点第3位まで
      |
      | 19/0416記
      | 値のＭＡＸ，ＭＩＮではないよ！
      | そのうち変えますが．
  APPS2_signal : Inport
  APPS2_Scope : Subsystem
  APPS2_signal_lowpass : Scope
  Divide : Product  Inputs=*/  RndMeth=Zero  SaturateOnIntegerOverflow=on
  Moving Average : dspstat3/Moving Average  Method=Sliding window  ForgettingFactorPort=off  SpecifyWindowLength=on  WindowLength=1000  ForgettingFactor=0.9  SimulateUsing=Code generation
  Sum1 : Sum  Inputs=|+-
  Sum3 : Sum  Inputs=-+
  Throttle2_MAX : Constant  Value=444  OutDataTypeStr=double
  Throttle2_MIN : Constant  Value=814  OutDataTypeStr=double
  Transfer Fcn : TransferFcn  Commented=on  Denominator=[1/(2*pi*5) 1]
  APPS2 : Outport  VectorParamsAs1DForOutWhenUnconnected=off
  wires:
  Moving Average/1 -> APPS2_signal_lowpass/1
  APPS2_signal/1 -> APPS2_Scope/1(In1), Sum1/1, Moving Average/1
  Divide/1 -> APPS2/1
  Throttle2_MAX/1 -> Sum3/2
  Sum1/1 -> Divide/1
  Sum3/1 -> Divide/2
  Throttle2_MIN/1 -> Sum1/2, Sum3/1

== system Driver_Input/Calibration3 ==
  note: 反時計回りが正
      | 時計回りが負
  SAS1_signal : Inport
  1/NuckleArmLength : Gain  Gain=1/72
  Add : Sum  Inputs=+-
  Asin : Trigonometry  Operator=asin
  Gain : Gain  Gain=-1
  SAS1_signal_0deg : Constant  Value=520
  Tielod mm/V : Gain  Gain=75/4
  Transfer Fcn : TransferFcn  Denominator=[1/(2*pi*5) 1]
  to Voltage : Gain  Gain=5/1023
  SAS1 : Outport  VectorParamsAs1DForOutWhenUnconnected=off
  wires:
  Gain/1 -> to Voltage/1
  to Voltage/1 -> Tielod mm/V/1  "Sensor Voltage"
  Asin/1 -> SAS1/1  "delta"
  Tielod mm/V/1 -> 1/NuckleArmLength/1  "Tielod Position"
  Transfer Fcn/1 -> Add/1
  1/NuckleArmLength/1 -> Asin/1  "sin(delta)"
  Add/1 -> Gain/1
  SAS1_signal_0deg/1 -> Add/2
  SAS1_signal/1 -> Transfer Fcn/1

== system Driver_Input/Calibration4 ==
  note: 反時計回りが正
      | 時計回りが負
  SAS2_signal : Inport
  1/NuckleArmLength : Gain  Gain=1/72
  Add : Sum  Inputs=+-
  Asin : Trigonometry  Operator=asin
  Gain : Gain  Gain=-1
  SAS1_signal_0deg : Constant  Value=440
  Tielod mm/V : Gain  Gain=75/5
  Transfer Fcn : TransferFcn  Denominator=[1/(2*pi*5) 1]
  to Voltage : Gain  Gain=5/1023
  SAS1 : Outport  VectorParamsAs1DForOutWhenUnconnected=off
  wires:
  Gain/1 -> to Voltage/1
  Add/1 -> Gain/1
  to Voltage/1 -> Tielod mm/V/1  "Sensor Voltage"
  Asin/1 -> SAS1/1  "delta"
  Tielod mm/V/1 -> 1/NuckleArmLength/1  "Tielod Position"
  Transfer Fcn/1 -> Add/1
  1/NuckleArmLength/1 -> Asin/1  "sin(delta)"
  SAS1_signal_0deg/1 -> Add/2
  SAS2_signal/1 -> Transfer Fcn/1

== system Driver_Input/Calibration5 ==
  BrakePressF_signal : Inport
  BrakePressF_Pa : Display
  Gain : Gain  Gain=1000
  MATLAB Function : MATLAB Function  TreatAsAtomicUnit=on
  Number to V : Gain  Gain=5/1023
  BrakePressF : Outport  VectorParamsAs1DForOutWhenUnconnected=off
  wires:
  MATLAB Function/1(bar) -> BrakePressF/1, BrakePressF_Pa/1
  BrakePressF_signal/1 -> Number to V/1
  Number to V/1 -> Gain/1
  Gain/1 -> MATLAB Function/1(mV)

== system Driver_Input/Calibration6 ==
  BrakePressR_signal : Inport
  10V to V : Gain  Gain=10
  BrakePressR_Pa : Display
  Gain : Gain  Gain=1000
  MATLAB Function : MATLAB Function  TreatAsAtomicUnit=on
  BrakePressR : Outport  VectorParamsAs1DForOutWhenUnconnected=off
  wires:
  MATLAB Function/1(bar) -> BrakePressR/1, BrakePressR_Pa/1
  10V to V/1 -> Gain/1
  Gain/1 -> MATLAB Function/1(mV)
  BrakePressR_signal/1 -> 10V to V/1

== system Driver_Input/Calibration7 ==
  note: キャリブレーション時
      | アクセルを踏んでいないときのAPPS value1の値を上に，
      | アクセル全開のときのAPPS value1の値を下に入れてね．
      | 小数点第3位まで
      |
      | 19/0416記
      | 値のＭＡＸ，ＭＩＮではないよ！
      | そのうち変えますが．
  BrakePressF_signal : Inport
  BrakePressF_MAX : Constant  Value=515  OutDataTypeStr=double
  BrakePressF_MIN : Constant  Value=826  OutDataTypeStr=double
  BrakePressF_Scope : Subsystem
  BrakePressF_signal_lowpass : Scope
  Divide : Product  Inputs=*/  RndMeth=Zero  SaturateOnIntegerOverflow=on
  Moving Average : dspstat3/Moving Average  Method=Sliding window  ForgettingFactorPort=off  SpecifyWindowLength=on  WindowLength=1000  ForgettingFactor=0.9  SimulateUsing=Code generation
  Sum1 : Sum  Inputs=|+-
  Sum3 : Sum  Inputs=-+
  BrakePressF : Outport  VectorParamsAs1DForOutWhenUnconnected=off
  wires:
  Moving Average/1 -> BrakePressF_signal_lowpass/1
  BrakePressF_signal/1 -> BrakePressF_Scope/1(BrakePressF_signal), Sum1/1, Moving Average/1
  Divide/1 -> BrakePressF/1
  BrakePressF_MAX/1 -> Sum3/2
  Sum1/1 -> Divide/1
  Sum3/1 -> Divide/2
  BrakePressF_MIN/1 -> Sum3/1, Sum1/2

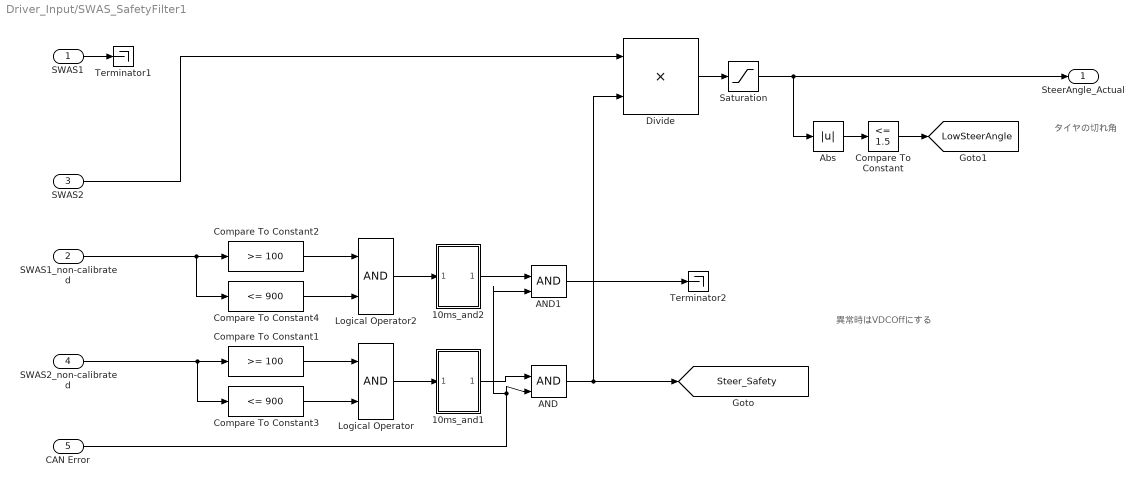
== system Driver_Input/SWAS_SafetyFilter1 ==
  note: タイヤの切れ角
  note: 異常時はVDCOffにする
  SWAS1 : Inport
  SWAS1_non-calibrated : Inport  Port=2
  SWAS2 : Inport  Port=3
  SWAS2_non-calibrated : Inport  Port=4
  CAN Error : Inport  Port=5
  10ms_and1 : Subsystem
  10ms_and2 : Subsystem
  AND : Logic  IconShape=distinctive  AllPortsSameDT=off  OutDataTypeStr=boolean
  AND1 : Logic  IconShape=distinctive  AllPortsSameDT=off  OutDataTypeStr=boolean
  Abs : Abs
  Compare To Constant : simulink/Logic and Bit Operations/Compare To Constant  relop=<=  const=1.5  OutDataTypeStr=boolean
  Compare To Constant1 : simulink/Logic and Bit Operations/Compare To Constant  relop=>=  const=100  OutDataTypeStr=boolean
  Compare To Constant2 : simulink/Logic and Bit Operations/Compare To Constant  relop=>=  const=100  OutDataTypeStr=boolean
  Compare To Constant3 : simulink/Logic and Bit Operations/Compare To Constant  relop=<=  const=900  OutDataTypeStr=boolean
  Compare To Constant4 : simulink/Logic and Bit Operations/Compare To Constant  relop=<=  const=900  OutDataTypeStr=boolean
  Divide : Product  Inputs=**
  Logical Operator : Logic  AllPortsSameDT=off  OutDataTypeStr=boolean
  Logical Operator2 : Logic  AllPortsSameDT=off  OutDataTypeStr=boolean
  Saturation : Saturate  UpperLimit=180  LowerLimit=-180
  Terminator1 : Terminator
  Terminator2 : Terminator
  SteerAngle_Actual : Outport  VectorParamsAs1DForOutWhenUnconnected=off
  tag scope: LowSteerAngle=global, Steer_Safety=global
  wires:
  SWAS1/1 -> Terminator1/1
  Compare To Constant/1 -> [LowSteerAngle]
  Abs/1 -> Compare To Constant/1
  10ms_and2/1(Out1) -> AND1/1
  Compare To Constant2/1 -> Logical Operator2/1
  Logical Operator2/1 -> 10ms_and2/1(In1)
  Compare To Constant4/1 -> Logical Operator2/2
  SWAS1_non-calibrated/1 -> Compare To Constant2/1, Compare To Constant4/1
  SWAS2/1 -> Divide/1
  10ms_and1/1(Out1) -> AND/1
  CAN Error/1 -> AND/2, AND1/2
  Saturation/1 -> Abs/1, SteerAngle_Actual/1
  Divide/1 -> Saturation/1
  AND1/1 -> Terminator2/1
  Compare To Constant3/1 -> Logical Operator/2
  SWAS2_non-calibrated/1 -> Compare To Constant1/1, Compare To Constant3/1
  Compare To Constant1/1 -> Logical Operator/1
  Logical Operator/1 -> 10ms_and1/1(In1)
  AND/1 -> Divide/2, [Steer_Safety]

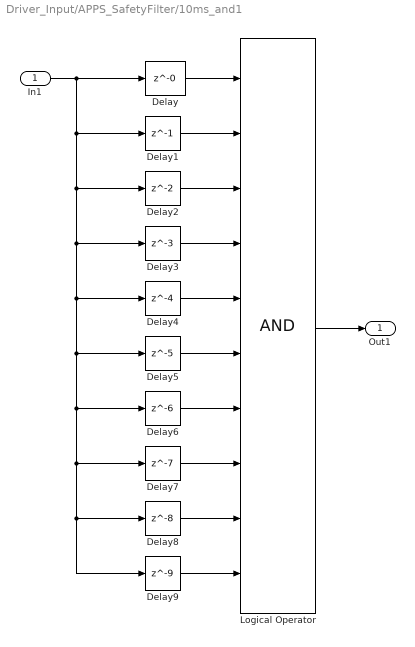
== system Driver_Input/APPS_SafetyFilter/10ms_and1 ==
  In1 : Inport
  Delay : Delay  DelayLength=0  InitialCondition=0
  Delay1 : Delay  DelayLength=1  InitialCondition=0
  Delay2 : Delay  InitialCondition=0
  Delay3 : Delay  DelayLength=3  InitialCondition=0
  Delay4 : Delay  DelayLength=4  InitialCondition=0
  Delay5 : Delay  DelayLength=5  InitialCondition=0
  Delay6 : Delay  DelayLength=6  InitialCondition=0
  Delay7 : Delay  DelayLength=7  InitialCondition=0
  Delay8 : Delay  DelayLength=8  InitialCondition=0
  Delay9 : Delay  DelayLength=9  InitialCondition=0
  Logical Operator : Logic  Inputs=10  AllPortsSameDT=off  OutDataTypeStr=boolean
  Out1 : Outport  VectorParamsAs1DForOutWhenUnconnected=off
  wires:
  Logical Operator/1 -> Out1/1
  Delay6/1 -> Logical Operator/7
  Delay7/1 -> Logical Operator/8
  Delay5/1 -> Logical Operator/6
  Delay9/1 -> Logical Operator/10
  Delay4/1 -> Logical Operator/5
  Delay3/1 -> Logical Operator/4
  Delay1/1 -> Logical Operator/2
  Delay/1 -> Logical Operator/1
  In1/1 -> Delay/1, Delay1/1, Delay2/1, Delay3/1, Delay4/1, Delay5/1, Delay6/1, Delay7/1, Delay8/1, Delay9/1
  Delay8/1 -> Logical Operator/9
  Delay2/1 -> Logical Operator/3

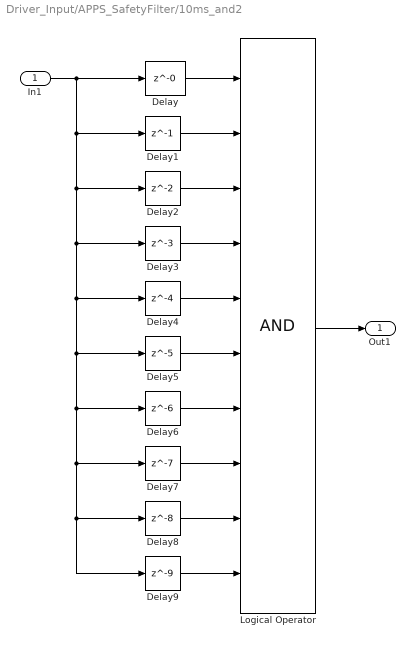
== system Driver_Input/APPS_SafetyFilter/10ms_and2 ==
  In1 : Inport
  Delay : Delay  DelayLength=0  InitialCondition=0
  Delay1 : Delay  DelayLength=1  InitialCondition=0
  Delay2 : Delay  InitialCondition=0
  Delay3 : Delay  DelayLength=3  InitialCondition=0
  Delay4 : Delay  DelayLength=4  InitialCondition=0
  Delay5 : Delay  DelayLength=5  InitialCondition=0
  Delay6 : Delay  DelayLength=6  InitialCondition=0
  Delay7 : Delay  DelayLength=7  InitialCondition=0
  Delay8 : Delay  DelayLength=8  InitialCondition=0
  Delay9 : Delay  DelayLength=9  InitialCondition=0
  Logical Operator : Logic  Inputs=10  AllPortsSameDT=off  OutDataTypeStr=boolean
  Out1 : Outport  VectorParamsAs1DForOutWhenUnconnected=off
  wires:
  Logical Operator/1 -> Out1/1
  Delay6/1 -> Logical Operator/7
  Delay7/1 -> Logical Operator/8
  Delay5/1 -> Logical Operator/6
  Delay9/1 -> Logical Operator/10
  Delay4/1 -> Logical Operator/5
  Delay3/1 -> Logical Operator/4
  Delay1/1 -> Logical Operator/2
  Delay/1 -> Logical Operator/1
  In1/1 -> Delay/1, Delay1/1, Delay2/1, Delay3/1, Delay4/1, Delay5/1, Delay6/1, Delay7/1, Delay8/1, Delay9/1
  Delay8/1 -> Logical Operator/9
  Delay2/1 -> Logical Operator/3

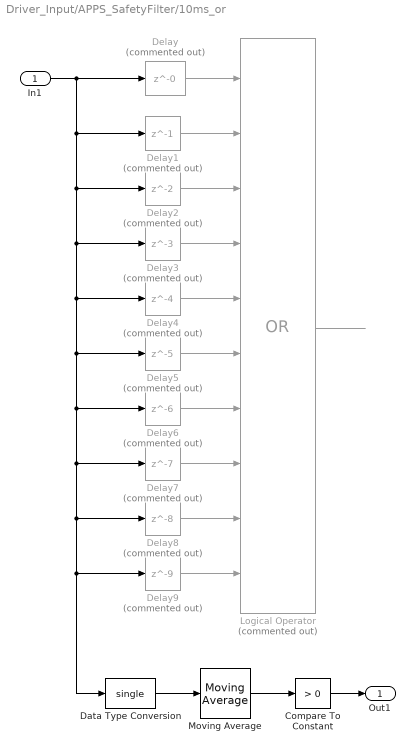
== system Driver_Input/APPS_SafetyFilter/10ms_or ==
  In1 : Inport
  Compare To Constant : simulink/Logic and Bit Operations/Compare To Constant  relop=>  const=0  OutDataTypeStr=boolean
  Data Type Conversion : DataTypeConversion  OutDataTypeStr=single
  Delay : Delay  Commented=on  DelayLength=0  InitialCondition=0
  Delay1 : Delay  Commented=on  DelayLength=1  InitialCondition=0
  Delay2 : Delay  Commented=on  InitialCondition=0
  Delay3 : Delay  Commented=on  DelayLength=3  InitialCondition=0
  Delay4 : Delay  Commented=on  DelayLength=4  InitialCondition=0
  Delay5 : Delay  Commented=on  DelayLength=5  InitialCondition=0
  Delay6 : Delay  Commented=on  DelayLength=6  InitialCondition=0
  Delay7 : Delay  Commented=on  DelayLength=7  InitialCondition=0
  Delay8 : Delay  Commented=on  DelayLength=8  InitialCondition=0
  Delay9 : Delay  Commented=on  DelayLength=9  InitialCondition=0
  Logical Operator : Logic  Commented=on  Operator=OR  Inputs=10  AllPortsSameDT=off  OutDataTypeStr=boolean
  Moving Average : dspstat3/Moving Average  Method=Sliding window  ForgettingFactorPort=off  SpecifyWindowLength=on  WindowLength=200  ForgettingFactor=0.9  SimulateUsing=Code generation
  Out1 : Outport  VectorParamsAs1DForOutWhenUnconnected=off
  wires:
  Data Type Conversion/1 -> Moving Average/1
  Compare To Constant/1 -> Out1/1
  Moving Average/1 -> Compare To Constant/1
  Logical Operator/1 -> ?
  Delay6/1 -> Logical Operator/7
  Delay7/1 -> Logical Operator/8
  Delay5/1 -> Logical Operator/6
  Delay9/1 -> Logical Operator/10
  Delay4/1 -> Logical Operator/5
  Delay3/1 -> Logical Operator/4
  Delay1/1 -> Logical Operator/2
  Delay/1 -> Logical Operator/1
  In1/1 -> Delay/1, Delay1/1, Delay2/1, Delay3/1, Delay4/1, Delay5/1, Delay6/1, Delay7/1, Delay8/1, Delay9/1, Data Type Conversion/1
  Delay8/1 -> Logical Operator/9
  Delay2/1 -> Logical Operator/3

== system Driver_Input/APPS_SafetyFilter/5ms_and ==
  In1 : Inport
  Delay : Delay  DelayLength=0  InitialCondition=0
  Delay1 : Delay  DelayLength=1  InitialCondition=0
  Delay2 : Delay  InitialCondition=0
  Delay3 : Delay  DelayLength=3  InitialCondition=0
  Delay4 : Delay  DelayLength=4  InitialCondition=0
  Logical Operator : Logic  Inputs=5  AllPortsSameDT=off  OutDataTypeStr=boolean
  Out1 : Outport  VectorParamsAs1DForOutWhenUnconnected=off
  wires:
  Logical Operator/1 -> Out1/1
  Delay4/1 -> Logical Operator/5
  Delay3/1 -> Logical Operator/4
  Delay1/1 -> Logical Operator/2
  Delay/1 -> Logical Operator/1
  In1/1 -> Delay/1, Delay1/1, Delay2/1, Delay3/1, Delay4/1
  Delay2/1 -> Logical Operator/3

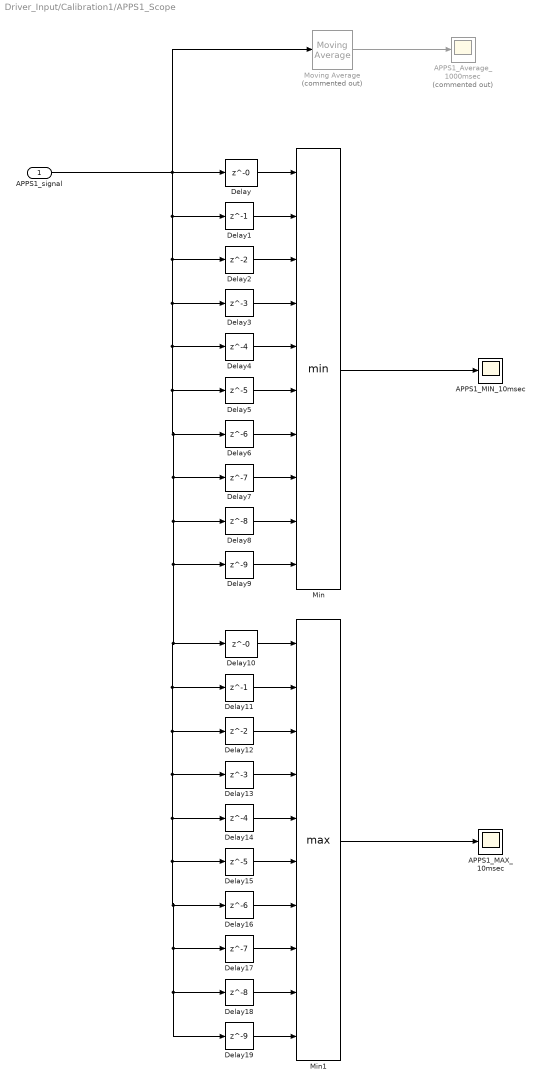
== system Driver_Input/Calibration1/APPS1_Scope ==
  APPS1_signal : Inport
  APPS1_Average_1000msec : Scope  Commented=on
  APPS1_MAX_10msec : Scope
  APPS1_MIN_10msec : Scope
  Delay : Delay  DelayLength=0  InitialCondition=0
  Delay1 : Delay  DelayLength=1  InitialCondition=0
  Delay10 : Delay  DelayLength=0  InitialCondition=0
  Delay11 : Delay  DelayLength=1  InitialCondition=0
  Delay12 : Delay  InitialCondition=0
  Delay13 : Delay  DelayLength=3  InitialCondition=0
  Delay14 : Delay  DelayLength=4  InitialCondition=0
  Delay15 : Delay  DelayLength=5  InitialCondition=0
  Delay16 : Delay  DelayLength=6  InitialCondition=0
  Delay17 : Delay  DelayLength=7  InitialCondition=0
  Delay18 : Delay  DelayLength=8  InitialCondition=0
  Delay19 : Delay  DelayLength=9  InitialCondition=0
  Delay2 : Delay  InitialCondition=0
  Delay3 : Delay  DelayLength=3  InitialCondition=0
  Delay4 : Delay  DelayLength=4  InitialCondition=0
  Delay5 : Delay  DelayLength=5  InitialCondition=0
  Delay6 : Delay  DelayLength=6  InitialCondition=0
  Delay7 : Delay  DelayLength=7  InitialCondition=0
  Delay8 : Delay  DelayLength=8  InitialCondition=0
  Delay9 : Delay  DelayLength=9  InitialCondition=0
  Min : MinMax  Inputs=10
  Min1 : MinMax  Function=max  Inputs=10
  Moving Average : dspstat3/Moving Average  Commented=on  Method=Sliding window  ForgettingFactorPort=off  SpecifyWindowLength=on  WindowLength=1000  ForgettingFactor=0.9  SimulateUsing=Code generation
  wires:
  APPS1_signal/1 -> Delay/1, Delay4/1, Delay7/1, Delay9/1, Delay10/1, Delay14/1, Delay17/1, Delay19/1, Delay18/1, Delay16/1, Delay15/1, Delay13/1, Delay12/1, Delay11/1, Delay8/1, Delay6/1, Delay5/1, Delay3/1, Delay2/1, Delay1/1, Moving Average/1
  Moving Average/1 -> APPS1_Average_1000msec/1
  Min1/1 -> APPS1_MAX_10msec/1
  Delay12/1 -> Min1/3
  Delay11/1 -> Min1/2
  Delay17/1 -> Min1/8
  Delay16/1 -> Min1/7
  Delay15/1 -> Min1/6
  Delay19/1 -> Min1/10
  Delay10/1 -> Min1/1
  Delay14/1 -> Min1/5
  Delay18/1 -> Min1/9
  Delay13/1 -> Min1/4
  Delay6/1 -> Min/7
  Delay7/1 -> Min/8
  Delay4/1 -> Min/5
  Delay3/1 -> Min/4
  Delay1/1 -> Min/2
  Delay8/1 -> Min/9
  Delay/1 -> Min/1
  Delay9/1 -> Min/10
  Delay2/1 -> Min/3
  Delay5/1 -> Min/6
  Min/1 -> APPS1_MIN_10msec/1

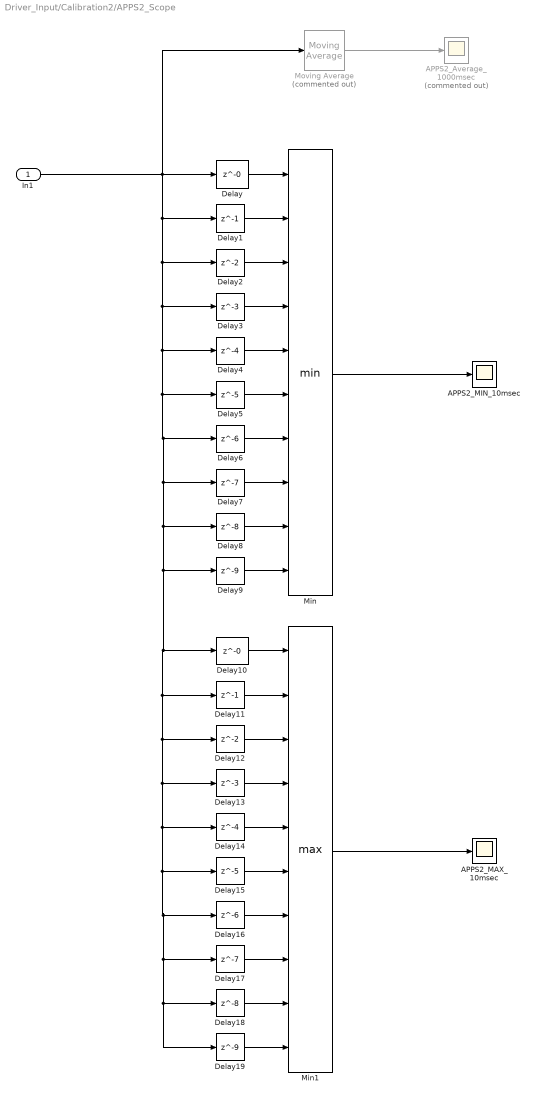
== system Driver_Input/Calibration2/APPS2_Scope ==
  In1 : Inport
  APPS2_Average_1000msec : Scope  Commented=on
  APPS2_MAX_10msec : Scope
  APPS2_MIN_10msec : Scope
  Delay : Delay  DelayLength=0  InitialCondition=0
  Delay1 : Delay  DelayLength=1  InitialCondition=0
  Delay10 : Delay  DelayLength=0  InitialCondition=0
  Delay11 : Delay  DelayLength=1  InitialCondition=0
  Delay12 : Delay  InitialCondition=0
  Delay13 : Delay  DelayLength=3  InitialCondition=0
  Delay14 : Delay  DelayLength=4  InitialCondition=0
  Delay15 : Delay  DelayLength=5  InitialCondition=0
  Delay16 : Delay  DelayLength=6  InitialCondition=0
  Delay17 : Delay  DelayLength=7  InitialCondition=0
  Delay18 : Delay  DelayLength=8  InitialCondition=0
  Delay19 : Delay  DelayLength=9  InitialCondition=0
  Delay2 : Delay  InitialCondition=0
  Delay3 : Delay  DelayLength=3  InitialCondition=0
  Delay4 : Delay  DelayLength=4  InitialCondition=0
  Delay5 : Delay  DelayLength=5  InitialCondition=0
  Delay6 : Delay  DelayLength=6  InitialCondition=0
  Delay7 : Delay  DelayLength=7  InitialCondition=0
  Delay8 : Delay  DelayLength=8  InitialCondition=0
  Delay9 : Delay  DelayLength=9  InitialCondition=0
  Min : MinMax  Inputs=10
  Min1 : MinMax  Function=max  Inputs=10
  Moving Average : dspstat3/Moving Average  Commented=on  Method=Sliding window  ForgettingFactorPort=off  SpecifyWindowLength=on  WindowLength=1000  ForgettingFactor=0.9  SimulateUsing=Code generation
  wires:
  Moving Average/1 -> APPS2_Average_1000msec/1
  In1/1 -> Delay/1, Delay4/1, Delay7/1, Delay9/1, Delay10/1, Delay14/1, Delay17/1, Delay19/1, Delay18/1, Delay16/1, Delay15/1, Delay13/1, Delay12/1, Delay11/1, Delay8/1, Delay6/1, Delay5/1, Delay3/1, Delay2/1, Delay1/1, Moving Average/1
  Min1/1 -> APPS2_MAX_10msec/1
  Delay12/1 -> Min1/3
  Delay11/1 -> Min1/2
  Delay17/1 -> Min1/8
  Delay16/1 -> Min1/7
  Delay15/1 -> Min1/6
  Delay19/1 -> Min1/10
  Delay10/1 -> Min1/1
  Delay14/1 -> Min1/5
  Delay18/1 -> Min1/9
  Delay13/1 -> Min1/4
  Delay6/1 -> Min/7
  Delay7/1 -> Min/8
  Delay4/1 -> Min/5
  Delay3/1 -> Min/4
  Delay1/1 -> Min/2
  Delay8/1 -> Min/9
  Delay/1 -> Min/1
  Delay9/1 -> Min/10
  Delay2/1 -> Min/3
  Delay5/1 -> Min/6
  Min/1 -> APPS2_MIN_10msec/1

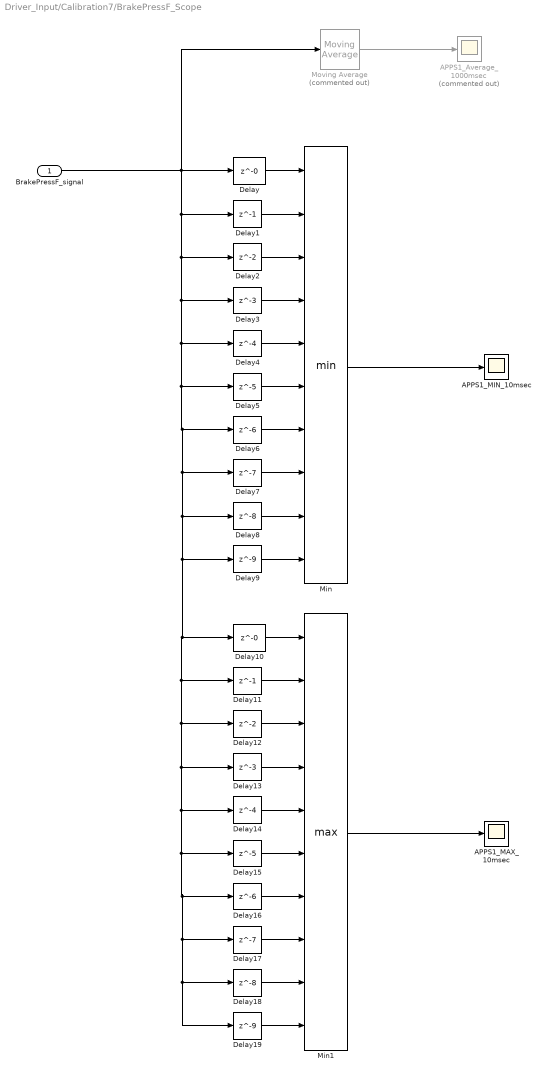
== system Driver_Input/Calibration7/BrakePressF_Scope ==
  BrakePressF_signal : Inport
  APPS1_Average_1000msec : Scope  Commented=on
  APPS1_MAX_10msec : Scope
  APPS1_MIN_10msec : Scope
  Delay : Delay  DelayLength=0  InitialCondition=0
  Delay1 : Delay  DelayLength=1  InitialCondition=0
  Delay10 : Delay  DelayLength=0  InitialCondition=0
  Delay11 : Delay  DelayLength=1  InitialCondition=0
  Delay12 : Delay  InitialCondition=0
  Delay13 : Delay  DelayLength=3  InitialCondition=0
  Delay14 : Delay  DelayLength=4  InitialCondition=0
  Delay15 : Delay  DelayLength=5  InitialCondition=0
  Delay16 : Delay  DelayLength=6  InitialCondition=0
  Delay17 : Delay  DelayLength=7  InitialCondition=0
  Delay18 : Delay  DelayLength=8  InitialCondition=0
  Delay19 : Delay  DelayLength=9  InitialCondition=0
  Delay2 : Delay  InitialCondition=0
  Delay3 : Delay  DelayLength=3  InitialCondition=0
  Delay4 : Delay  DelayLength=4  InitialCondition=0
  Delay5 : Delay  DelayLength=5  InitialCondition=0
  Delay6 : Delay  DelayLength=6  InitialCondition=0
  Delay7 : Delay  DelayLength=7  InitialCondition=0
  Delay8 : Delay  DelayLength=8  InitialCondition=0
  Delay9 : Delay  DelayLength=9  InitialCondition=0
  Min : MinMax  Inputs=10
  Min1 : MinMax  Function=max  Inputs=10
  Moving Average : dspstat3/Moving Average  Commented=on  Method=Sliding window  ForgettingFactorPort=off  SpecifyWindowLength=on  WindowLength=1000  ForgettingFactor=0.9  SimulateUsing=Code generation
  wires:
  BrakePressF_signal/1 -> Delay/1, Delay4/1, Delay7/1, Delay9/1, Delay10/1, Delay14/1, Delay17/1, Delay19/1, Delay18/1, Delay16/1, Delay15/1, Delay13/1, Delay12/1, Delay11/1, Delay8/1, Delay6/1, Delay5/1, Delay3/1, Delay2/1, Delay1/1, Moving Average/1
  Moving Average/1 -> APPS1_Average_1000msec/1
  Min1/1 -> APPS1_MAX_10msec/1
  Delay12/1 -> Min1/3
  Delay11/1 -> Min1/2
  Delay17/1 -> Min1/8
  Delay16/1 -> Min1/7
  Delay15/1 -> Min1/6
  Delay19/1 -> Min1/10
  Delay10/1 -> Min1/1
  Delay14/1 -> Min1/5
  Delay18/1 -> Min1/9
  Delay13/1 -> Min1/4
  Delay6/1 -> Min/7
  Delay7/1 -> Min/8
  Delay4/1 -> Min/5
  Delay3/1 -> Min/4
  Delay1/1 -> Min/2
  Delay8/1 -> Min/9
  Delay/1 -> Min/1
  Delay9/1 -> Min/10
  Delay2/1 -> Min/3
  Delay5/1 -> Min/6
  Min/1 -> APPS1_MIN_10msec/1

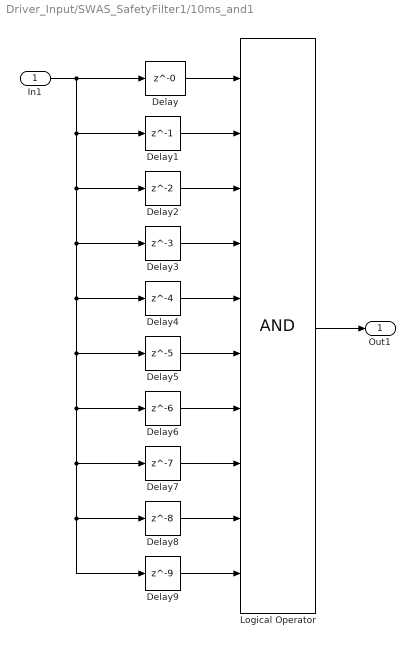
== system Driver_Input/SWAS_SafetyFilter1/10ms_and1 ==
  In1 : Inport
  Delay : Delay  DelayLength=0  InitialCondition=0
  Delay1 : Delay  DelayLength=1  InitialCondition=0
  Delay2 : Delay  InitialCondition=0
  Delay3 : Delay  DelayLength=3  InitialCondition=0
  Delay4 : Delay  DelayLength=4  InitialCondition=0
  Delay5 : Delay  DelayLength=5  InitialCondition=0
  Delay6 : Delay  DelayLength=6  InitialCondition=0
  Delay7 : Delay  DelayLength=7  InitialCondition=0
  Delay8 : Delay  DelayLength=8  InitialCondition=0
  Delay9 : Delay  DelayLength=9  InitialCondition=0
  Logical Operator : Logic  Inputs=10  AllPortsSameDT=off  OutDataTypeStr=boolean
  Out1 : Outport  VectorParamsAs1DForOutWhenUnconnected=off
  wires:
  Delay2/1 -> Logical Operator/3
  Delay8/1 -> Logical Operator/9
  In1/1 -> Delay9/1, Delay8/1, Delay7/1, Delay6/1, Delay5/1, Delay4/1, Delay3/1, Delay2/1, Delay1/1, Delay/1
  Delay/1 -> Logical Operator/1
  Delay1/1 -> Logical Operator/2
  Delay3/1 -> Logical Operator/4
  Delay4/1 -> Logical Operator/5
  Delay9/1 -> Logical Operator/10
  Delay5/1 -> Logical Operator/6
  Delay7/1 -> Logical Operator/8
  Delay6/1 -> Logical Operator/7
  Logical Operator/1 -> Out1/1
